simulink model "Lab5simu"  (R2018a)
settings: Solver=VariableStepAuto  StartTime=0.0  StopTime=10.0  MaxStep=0.001  RelTol=1e-3
values from neighbouring files (symbols this model uses):
  Wn = 4    [Lab5.m]
  xi = Xi(i)    [Lab5.m]
settings Model: Creator=aplov  LastModifiedBy=aplov

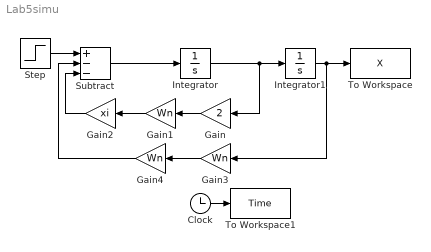
== system Lab5simu ==
  Clock : Clock
  Gain : Gain  Gain=2
  Gain1 : Gain  Gain=Wn
  Gain2 : Gain  Gain=xi
  Gain3 : Gain  Gain=Wn
  Gain4 : Gain  Gain=Wn
  Integrator : Integrator
  Integrator1 : Integrator
  Step : Step  Time=0.1  SampleTime=0
  Subtract : Sum  Inputs=+--
  To Workspace : ToWorkspace  VariableName=X  SampleTime=-1
  To Workspace1 : ToWorkspace  VariableName=Time  SampleTime=-1
  wires:
  Step/1 -> Subtract/1
  Subtract/1 -> Integrator/1
  Integrator/1 -> Gain/1, Integrator1/1
  Integrator1/1 -> Gain3/1, To Workspace/1
  Gain/1 -> Gain1/1
  Gain1/1 -> Gain2/1
  Gain3/1 -> Gain4/1
  Gain4/1 -> Subtract/2
  Gain2/1 -> Subtract/3
  Clock/1 -> To Workspace1/1
